simulink model "PV_ObservadorPerturbacion"  (R2018b)
settings: Solver=VariableStepAuto  StartTime=0.0  StopTime=10.0  RelTol=1e-3
undefined symbols (not defined in the file): AHat, BHat, CHat, DHat, EEd, EEdObs, FHat, K, Kgain, kgainObs, Tao
settings Model: Creator=AlfredoMaussa  LastModifiedBy=AlfredoMaussa

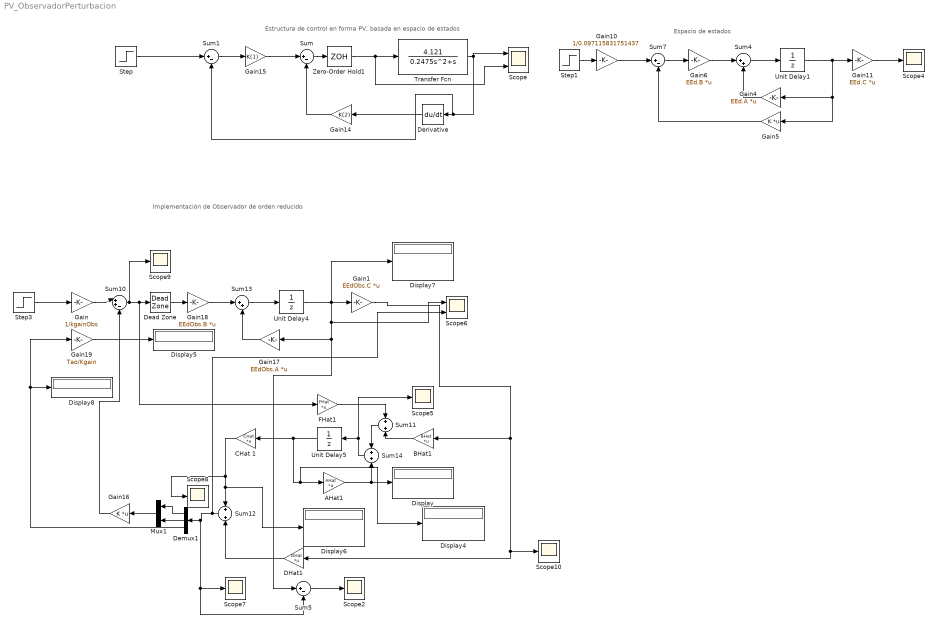
== system PV_ObservadorPerturbacion ==
  note: Implementación de Observador de orden reducido
  note: Estructura de control en forma PV, basada en espacio de estados
  note: Espacio de estados
  AHat1 : Gain  Gain=AHat  Multiplication=Matrix(K*u)
  BHat1 : Gain  Gain=BHat  Multiplication=Matrix(K*u)
  CHat 1 : Gain  Gain=CHat  Multiplication=Matrix(K*u)
  DHat1 : Gain  Gain=DHat  Multiplication=Matrix(K*u)
  Dead Zone : DeadZone  LowerValue=0  UpperValue=0  SaturateOnIntegerOverflow=on
  Demux1 : Demux  Outputs=3
  Derivative : Derivative  CoefficientInTFapproximation=100
  Display{,4..8} (6 alike) : Display
  FHat1 : Gain  Gain=FHat  Multiplication=Matrix(K*u)
  Gain : Gain  Gain=1/kgainObs
  Gain1 : Gain  Gain=EEdObs.C  Multiplication=Matrix(K*u)
  Gain10 : Gain  Gain=1/0.097115831751437
  Gain11 : Gain  Gain=EEd.C  Multiplication=Matrix(K*u)
  Gain14 : Gain  Gain=K(2)
  Gain15 : Gain  Gain=K(1)
  Gain16 : Gain  Gain=K  Multiplication=Matrix(K*u)
  Gain17 : Gain  Gain=EEdObs.A  Multiplication=Matrix(K*u)
  Gain18 : Gain  Gain=EEdObs.B  Multiplication=Matrix(K*u)
  Gain19 : Gain  Gain=Tao/Kgain
  Gain4 : Gain  Gain=EEd.A  Multiplication=Matrix(K*u)
  Gain5 : Gain  Gain=K  Multiplication=Matrix(K*u)
  Gain6 : Gain  Gain=EEd.B  Multiplication=Matrix(K*u)
  Mux1 : Mux  Inputs=2
  Scope : Scope  NumInputPorts=2
  Scope{2,4..5,7..10} (7 alike) : Scope
  Scope6 : Scope  NumInputPorts=2
  Step : Step  Time=0  SampleTime=0
  Step1 : Step  Time=0  SampleTime=0
  Step3 : Step  Time=0  SampleTime=0
  Sum{,1,5,7} (4 alike) : Sum  Inputs=|+-
  Sum10 : Sum  Inputs=|++-
  Sum11 : Sum  Inputs=+|+
  Sum12 : Sum  Inputs=+||+
  Sum13 : Sum  Inputs=|++
  Sum14 : Sum  Inputs=+|+
  Sum4 : Sum  Inputs=|++
  Transfer Fcn : TransferFcn  Numerator=[4.121]  Denominator=[0.2475 1 0]
  Unit Delay1 : UnitDelay  SampleTime=0.005
  Unit Delay4 : UnitDelay  InitialCondition=[0,0,15]  SampleTime=0.005
  Unit Delay5 : UnitDelay  InitialCondition=[0,0]  SampleTime=0.005
  Zero-Order Hold1 : ZeroOrderHold  SampleTime=0.005
  wires:
  Gain15/1 -> Sum/1
  Mux1/1 -> Gain16/1
  CHat 1/1 -> Sum12/1, Display6/1, Scope8/1
  Gain/1 -> Sum10/1
  Unit Delay5/1 -> CHat 1/1, Display4/1, AHat1/1
  Gain10/1 -> Sum7/1
  Sum11/1 -> Sum14/1
  Gain6/1 -> Sum4/1
  Sum13/1 -> Unit Delay4/1
  FHat1/1 -> Sum11/1
  Sum4/1 -> Unit Delay1/1
  Sum10/1 -> Scope9/1, FHat1/1, Dead Zone/1
  BHat1/1 -> Sum11/2
  Unit Delay4/1 -> Display7/1, Scope6/1, Sum5/1, Gain17/1, Gain1/1
  Gain18/1 -> Sum13/1
  Gain17/1 -> Sum13/2
  Gain11/1 -> Scope4/1
  Sum14/1 -> Scope5/1, Unit Delay5/1
  DHat1/1 -> Sum12/2
  Gain1/1 -> DHat1/1, Scope10/1, BHat1/1
  Derivative/1 -> Gain14/1
  Sum1/1 -> Gain15/1
  Gain4/1 -> Sum4/2
  Sum12/1 -> Scope6/2, Sum5/2, Scope7/1, Demux1/1
  Step1/1 -> Gain10/1
  Unit Delay1/1 -> Gain11/1, Gain5/1, Gain4/1
  Demux1/1 -> Mux1/1
  Step/1 -> Sum1/1
  Sum/1 -> Zero-Order Hold1/1
  Gain5/1 -> Sum7/2
  Demux1/2 -> Mux1/2
  Sum7/1 -> Gain6/1
  Step3/1 -> Gain/1
  Gain14/1 -> Sum/2
  Transfer Fcn/1 -> Sum1/2, Derivative/1, Scope/1
  AHat1/1 -> Sum14/2, Display/1
  Zero-Order Hold1/1 -> Scope/2, Transfer Fcn/1
  Dead Zone/1 -> Gain18/1
  Demux1/3 -> Display8/1, Gain19/1
  Gain19/1 -> Display5/1
  Sum5/1 -> Scope2/1
  Gain16/1 -> Sum10/3
